simulink model "hough_only"  (R2020a)
settings: Solver=VariableStepAuto  StartTime=0.0  StopTime=10.0  RelTol=1e-3
values from neighbouring files (symbols this model uses):
  maxRho = ceil(sqrt((height/2)^2+(width/2)^2))    [setup.m]
libraries: library x4
settings Model: Creator=david  LastModifiedBy=david

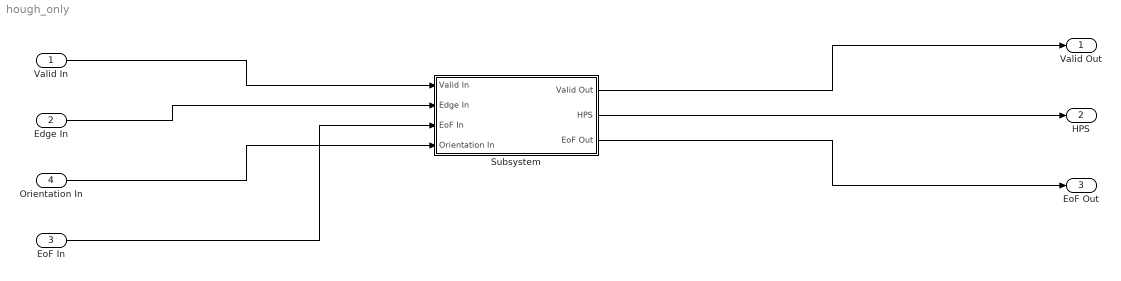
== system hough_only ==
  Valid In : Inport
  Edge In : Inport  Port=2
  EoF In : Inport  Port=3
  Orientation In : Inport  Port=4
  Subsystem : Subsystem
  Valid Out : Outport  VectorParamsAs1DForOutWhenUnconnected=off
  HPS : Outport  Port=2  VectorParamsAs1DForOutWhenUnconnected=off
  EoF Out : Outport  Port=3  VectorParamsAs1DForOutWhenUnconnected=off
  wires:
  Valid In/1 -> Subsystem/1(Valid In)
  Edge In/1 -> Subsystem/2(Edge In)
  EoF In/1 -> Subsystem/3(EoF In)
  Orientation In/1 -> Subsystem/4(Orientation In)
  Subsystem/1(Valid Out) -> Valid Out/1
  Subsystem/2(HPS) -> HPS/1
  Subsystem/3(EoF Out) -> EoF Out/1

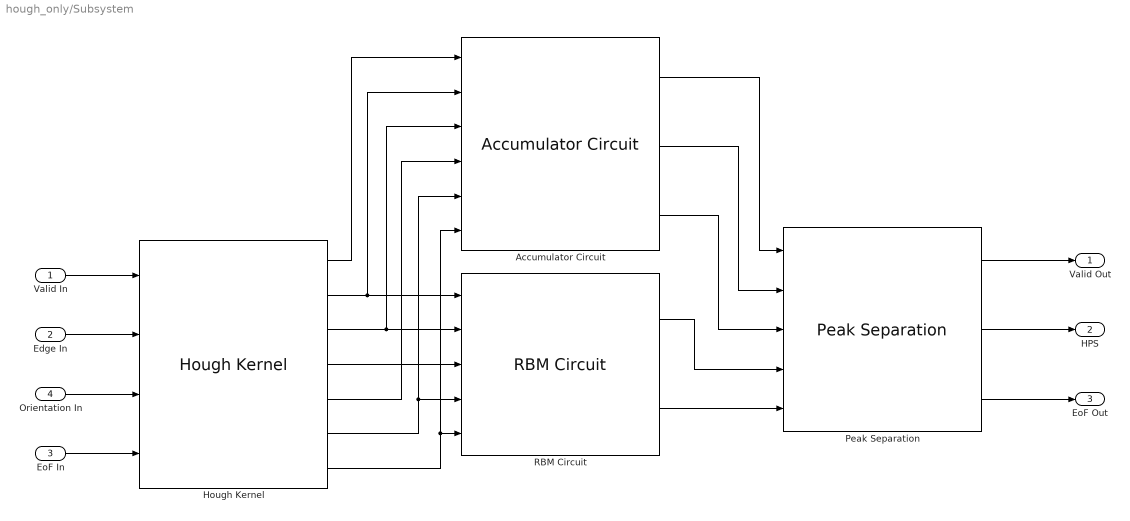
== system hough_only/Subsystem ==
  Valid In : Inport
  Edge In : Inport  Port=2
  EoF In : Inport  Port=3
  Orientation In : Inport  Port=4
  Accumulator Circuit : library/Accumulator Circuit  height=height  width=width  rhoBits=ceil(log2(maxRho*2))  nTheta=nTheta  nRho=nRho
  Hough Kernel : library/Hough Kernel  rhoBits=ceil(log2(maxRho*2))  height=height  width=width  dTheta=1
  Peak Separation : library/Peak Separation  nRho=nRho  nTheta=nTheta
  RBM Circuit : library/RBM Circuit  height=height  width=width  nTheta=nTheta  rhoBits=ceil(log2(maxRho*2))  nRho=nRho
  Valid Out : Outport  VectorParamsAs1DForOutWhenUnconnected=off
  HPS : Outport  Port=2  VectorParamsAs1DForOutWhenUnconnected=off
  EoF Out : Outport  Port=3  VectorParamsAs1DForOutWhenUnconnected=off
  wires:
  Accumulator Circuit/2 -> Peak Separation/2
  Edge In/1 -> Hough Kernel/2
  Hough Kernel/4 -> RBM Circuit/3
  Hough Kernel/1 -> Accumulator Circuit/1
  Valid In/1 -> Hough Kernel/1
  Hough Kernel/3 -> Accumulator Circuit/3, RBM Circuit/2
  EoF In/1 -> Hough Kernel/4
  Orientation In/1 -> Hough Kernel/3
  RBM Circuit/2 -> Peak Separation/5
  Hough Kernel/5 -> Accumulator Circuit/4
  Hough Kernel/2 -> Accumulator Circuit/2, RBM Circuit/1
  Hough Kernel/6 -> Accumulator Circuit/5, RBM Circuit/4
  Hough Kernel/7 -> Accumulator Circuit/6, RBM Circuit/5
  Peak Separation/2 -> HPS/1
  Peak Separation/3 -> EoF Out/1
  RBM Circuit/1 -> Peak Separation/4
  Peak Separation/1 -> Valid Out/1
  Accumulator Circuit/1 -> Peak Separation/1
  Accumulator Circuit/3 -> Peak Separation/3
